simulink model "powerconnection"  (R2023a)
settings: Solver=VariableStepAuto  StartTime=0.0  StopTime=8  RelTol=1e-3
libraries: spsBreakerLib x3, spsACVoltageSourceLib x2, spsSeriesRLCBranchLib x2, spsSeriesRLCLoadLib x2, spsCurrentMeasurementLib x1, dspstat3 x1, spsVoltageMeasurementLib x1, sps_lib x1
settings Model: Creator=Renjit Manoj VJ  LastModifiedBy=Renjit Manoj VJ

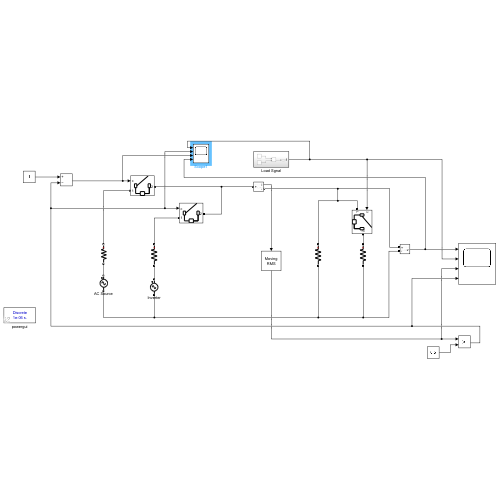
[thumbnail: Simulink's stored preview of the top-level diagram]
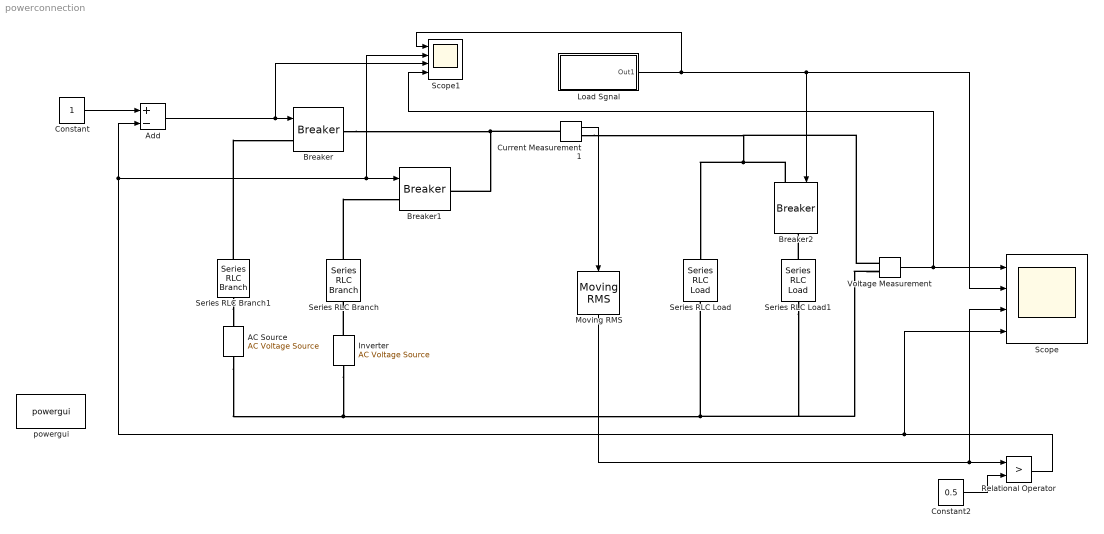
== system powerconnection ==
  AC Source : spsACVoltageSourceLib/AC Voltage Source  Amplitude=325  Phase=0  Frequency=50  SampleTime=0  Measurements=None  BusType=swing  Pref=10e3  Qref=0  Qmin=-inf  Qmax=+inf
  Add : Sum  Inputs=+-
  Breaker : spsBreakerLib/Breaker  InitialState=0  SwitchingTimes="[1/60  5/60]"  External=on  BreakerResistance=0.01  SnubberResistance=1e6  SnubberCapacitance=inf  Measurements=None  MoreParameters=on  NoBreakLoop=off
  Breaker1 : spsBreakerLib/Breaker  InitialState=0  SwitchingTimes="[1/60  5/60]"  External=on  BreakerResistance=0.01  SnubberResistance=1e6  SnubberCapacitance=inf  Measurements=None  MoreParameters=on  NoBreakLoop=off
  Breaker2 : spsBreakerLib/Breaker  InitialState=0  SwitchingTimes="[1/60  5/60]"  External=on  BreakerResistance=0.01  SnubberResistance=1e6  SnubberCapacitance=inf  Measurements=None  MoreParameters=on  NoBreakLoop=off
  Constant : Constant
  Constant2 : Constant  Value=0.5
  Current Measurement1 : spsCurrentMeasurementLib/Current Measurement  PhasorSimulation=off  OutputType=Complex  PSBequivalent=0
  Inverter : spsACVoltageSourceLib/AC Voltage Source  Amplitude=325  Phase=0  Frequency=50  SampleTime=0  Measurements=None  BusType=swing  Pref=10e3  Qref=0  Qmin=-inf  Qmax=+inf
  Load Sgnal : Subsystem
  Moving RMS : dspstat3/Moving RMS  Method=Sliding window  ForgettingFactorPort=off  SpecifyWindowLength=off  WindowLength=4  OverlapLength=3  AllowArbitraryInputLength=off  ForgettingFactor=0.9  SimulateUsing=Code generation
  Relational Operator : RelationalOperator  Operator=>  OutDataTypeStr=boolean  RndMeth=Simplest  InputSameDT=off
  Scope : Scope  NumInputPorts=4
  Scope1 : Scope  NumInputPorts=4
  Series RLC Branch : spsSeriesRLCBranchLib/Series RLC Branch  LConnTagsString=__new0  RConnTagsString=__new0  BranchType=R  Resistance=1  Inductance=1e-3  SetiL0=off  InitialCurrent=0  Capacitance=1e-6  Setx0=off  InitialVoltage=0  Measurements=None
  Series RLC Branch1 : spsSeriesRLCBranchLib/Series RLC Branch  LConnTagsString=__new0  RConnTagsString=__new0  BranchType=R  Resistance=100  Inductance=1e-3  SetiL0=off  InitialCurrent=0  Capacitance=1e-6  Setx0=off  InitialVoltage=0  Measurements=None
  Series RLC Load : spsSeriesRLCLoadLib/Series RLC Load  LConnTagsString=a  RConnTagsString=__new0  NominalVoltage=230  NominalFrequency=50  ActivePower=100  InductivePower=0  CapacitivePower=0  Setx0=off  InitialVoltage=0  SetiL0=off  InitialCurrent=0  Measurements=None  LoadType=constant Z
  Series RLC Load1 : spsSeriesRLCLoadLib/Series RLC Load  LConnTagsString=a  RConnTagsString=__new0  NominalVoltage=230  NominalFrequency=50  ActivePower=100  InductivePower=0  CapacitivePower=0  Setx0=off  InitialVoltage=0  SetiL0=off  InitialCurrent=0  Measurements=None  LoadType=constant Z
  Voltage Measurement : spsVoltageMeasurementLib/Voltage Measurement  PhasorSimulation=off  OutputType=Complex  PSBequivalent=0
  powergui : sps_lib/powergui  Priority=1  SimulationMode=Discrete  SampleTime=1e-6  frequency=60  Iterations=50  frequencyindice=50  Pbase=100e6  ErrMax=1e-4  UnitsV=kV  UnitsW=MW  buscounter=0  FunctionMessages=off  echomessages=off  EnableUseOfTLC=off  CurrentSourceSwitches=off  DisableSnubberDevices=off  DisableRonSwitches=off  DisableVfSwitches=off  DisplayEquations=off  AutomaticDiscreteSolvers=off  SolverType=Tustin/Backward Euler (TBE)  Interpol=off  ExternalGateDelay=off  methode=off  Ts=100  x0status=blocks  SPID=on  SwTol=0  HookPort=off  NonlinearTolerance=1e-4  nMaxIteration=100  ContinueOnMaxIteration=off  RestoreLinks=warning  ResistiveCurrentMeasurement=off  Frange=[0:2:500]  Ylog=off  Xlog=on  ShowGrid=off  save=off  variable=ZData  structure=0  ZoomFFT=off  StartTime=0.0  cycles=1  DisplayStyle=1  fundamental=60  FreqAxis=off  MaxFrequency=1000  frequencyindicesteady=1  RmsSteady=1  display=off
  wires:
  Voltage Measurement/1 -> Scope1/4, Scope/1
  Constant/1 -> Add/1
  Add/1 -> Scope1/3, Breaker/1
  Current Measurement1/1 -> Moving RMS/1
  Constant2/1 -> Relational Operator/2
  Moving RMS/1 -> Scope/3, Relational Operator/1
  Relational Operator/1 -> Scope/4, Add/2, Scope1/2, Breaker1/1
  Load Sgnal/1(Out1) -> Scope/2, Breaker2/1, Scope1/1
  connections:
  AC Source/LConn1 -- Inverter/LConn1 -- Voltage Measurement/LConn2 -- Series RLC Load1/RConn1 -- Series RLC Load/RConn1
  Inverter/RConn1 -- Series RLC Branch/RConn1
  Series RLC Branch1/RConn1 -- AC Source/RConn1
  Current Measurement1/LConn1 -- Breaker/RConn1 -- Breaker1/RConn1
  Series RLC Load1/LConn1 -- Breaker2/RConn1
  Breaker2/LConn1 -- Series RLC Load/LConn1 -- Current Measurement1/RConn1 -- Voltage Measurement/LConn1
  Series RLC Branch/LConn1 -- Breaker1/LConn1
  Series RLC Branch1/LConn1 -- Breaker/LConn1

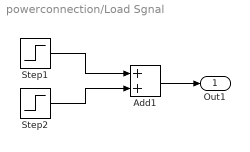
== system powerconnection/Load Sgnal ==
  Add1 : Sum
  Step1 : Step  Time=0.4  SampleTime=0
  Step2 : Step  Time=1.4  After=-1  SampleTime=0
  Out1 : Outport
  wires:
  Step1/1 -> Add1/1
  Add1/1 -> Out1/1
  Step2/1 -> Add1/2
